simulink model "discrete_model"  (R2018a)
settings: Solver=VariableStepAuto  StartTime=0.0  StopTime=24*60*60  RelTol=1e-3
values from neighbouring files (symbols this model uses):
  alpha = 0.05    [init.m]
  C_T = 12000    [init.m]
  epsilon = 5e-5    (= 5e-05)    [init.m]
  k_N = 2e-4    (= 0.0002)    [init.m]
  k_T = 20    [init.m]
  L0 = 1    [init.m]
  L_opt = 10    [init.m]
  N0 = 1    [init.m]
  N_opt = 150    [init.m]
  q_p = 0.002    [init.m]
  T0 = 20    [init.m]
  T_opt = 22    [init.m]
  T_sample = 1    [init.m]
libraries: simulink x2
settings Model: Creator=Mahsa  LastModifiedBy=Mahsa

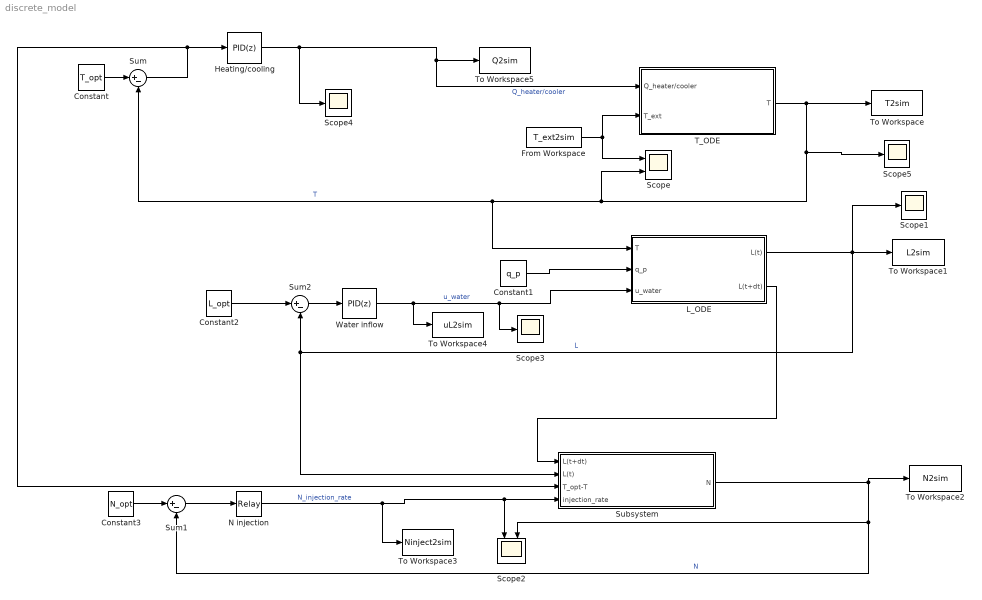
== system discrete_model ==
  Constant : Constant  Value=T_opt
  Constant1 : Constant  Value=q_p
  Constant2 : Constant  Value=L_opt
  Constant3 : Constant  Value=N_opt
  From Workspace : FromWorkspace  VariableName=T_ext2sim  SampleTime=0
  "Heating/cooling " : simulink/Continuous/PID Controller  Controller=PID  TimeDomain=Discrete-time  SampleTime=T_sample  IntegratorMethod=Forward Euler  FilterMethod=Forward Euler  Form=Parallel  UseFilter=on  ControllerParametersSource=internal  P=26.6328130643636  I=0.0891686910196959  D=-511.482477785438  N=0.00506771888250834  InitialConditionSource=internal  InitialConditionForIntegrator=0  InitialConditionForFilter=0  ExternalReset=none  LimitOutput=off  UpperSaturationLimit=inf  LowerSaturationLimit=-inf  LinearizeAsGain=on  AntiWindupMode=none  Kb=1  TrackingMode=off  Kt=1  PParamMin=[]  PParamMax=[]  IParamMin=[]  IParamMax=[]  DParamMin=[]  DParamMax=[]  NParamMin=[]  NParamMax=[]  KbParamMin=[]  KbParamMax=[]  KtParamMin=[]  KtParamMax=[]  POutMin=[]  POutMax=[]  IOutMin=[]  IOutMax=[]  DOutMin=[]  DOutMax=[]  NOutMin=[]  NOutMax=[]  KbOutMin=[]  KbOutMax=[]  KtOutMin=[]  KtOutMax=[]  IntegratorOutMin=[]  IntegratorOutMax=[]  FilterOutMin=[]  FilterOutMax=[]  SumOutMin=[]  SumOutMax=[]  SumI1OutMin=[]  SumI1OutMax=[]  SumI2OutMin=[]  SumI2OutMax=[]  SumI3OutMin=[]  SumI3OutMax=[]  SumDOutMin=[]  SumDOutMax=[]  SaturationOutMin=[]  SaturationOutMax=[]  IntegratorContinuousStateAttributes=''  IntegratorStateMustResolveToSignalObject=off  IntegratorRTWStateStorageClass=Auto  FilterContinuousStateAttributes=''  FilterStateMustResolveToSignalObject=off  FilterRTWStateStorageClass=Auto  DifferentiatorICPrevScaledInput=0  DifferentiatorOutMin=[]  DifferentiatorOutMax=[]  FilterDiffOutCoefMin=[]  FilterDiffOutCoefMax=[]  SumDenOutMin=[]  SumDenOutMax=[]  SumNumOutMin=[]  SumNumOutMax=[]  ReciprocalOutMin=[]  ReciprocalOutMax=[]  DivideOutMin=[]  DivideOutMax=[]  TunerSelectOption=Transfer Function Based (PID Tuner App)
  L_ODE : Subsystem
  N injection : Relay  OnSwitchValue=50  OffSwitchValue=-50  OnOutputValue=R
  Scope : Scope  NumInputPorts=2
  Scope{1,3..5} (4 alike) : Scope
  Scope2 : Scope  NumInputPorts=2
  Subsystem : Subsystem
  Sum : Sum  Inputs=|+-
  Sum1 : Sum  Inputs=|+-
  Sum2 : Sum  Inputs=|+-
  T_ODE : Subsystem
  To Workspace : ToWorkspace  VariableName=T2sim  SaveFormat=Timeseries  SampleTime=T_sample
  To Workspace1 : ToWorkspace  VariableName=L2sim  SaveFormat=Timeseries  SampleTime=T_sample
  To Workspace2 : ToWorkspace  VariableName=N2sim  SaveFormat=Timeseries  SampleTime=T_sample
  To Workspace3 : ToWorkspace  VariableName=Ninject2sim  SaveFormat=Timeseries  SampleTime=T_sample
  To Workspace4 : ToWorkspace  VariableName=uL2sim  SaveFormat=Timeseries  SampleTime=T_sample
  To Workspace5 : ToWorkspace  VariableName=Q2sim  SaveFormat=Timeseries  SampleTime=T_sample
  Water inflow : simulink/Continuous/PID Controller  Controller=PID  TimeDomain=Discrete-time  SampleTime=T_sample  IntegratorMethod=Forward Euler  FilterMethod=Forward Euler  Form=Parallel  UseFilter=on  ControllerParametersSource=internal  P=0.028808901415482  I=0.000153529168152366  D=-0.200332739399639  N=0.0470716938872077  InitialConditionSource=internal  InitialConditionForIntegrator=0  InitialConditionForFilter=0  ExternalReset=none  LimitOutput=on  UpperSaturationLimit=inf  LowerSaturationLimit=0  LinearizeAsGain=on  AntiWindupMode=none  Kb=1  TrackingMode=off  Kt=1  PParamMin=[]  PParamMax=[]  IParamMin=[]  IParamMax=[]  DParamMin=[]  DParamMax=[]  NParamMin=[]  NParamMax=[]  KbParamMin=[]  KbParamMax=[]  KtParamMin=[]  KtParamMax=[]  POutMin=[]  POutMax=[]  IOutMin=[]  IOutMax=[]  DOutMin=[]  DOutMax=[]  NOutMin=[]  NOutMax=[]  KbOutMin=[]  KbOutMax=[]  KtOutMin=[]  KtOutMax=[]  IntegratorOutMin=[]  IntegratorOutMax=[]  FilterOutMin=[]  FilterOutMax=[]  SumOutMin=[]  SumOutMax=[]  SumI1OutMin=[]  SumI1OutMax=[]  SumI2OutMin=[]  SumI2OutMax=[]  SumI3OutMin=[]  SumI3OutMax=[]  SumDOutMin=[]  SumDOutMax=[]  SaturationOutMin=[]  SaturationOutMax=[]  IntegratorContinuousStateAttributes=''  IntegratorStateMustResolveToSignalObject=off  IntegratorRTWStateStorageClass=Auto  FilterContinuousStateAttributes=''  FilterStateMustResolveToSignalObject=off  FilterRTWStateStorageClass=Auto  DifferentiatorICPrevScaledInput=0  DifferentiatorOutMin=[]  DifferentiatorOutMax=[]  FilterDiffOutCoefMin=[]  FilterDiffOutCoefMax=[]  SumDenOutMin=[]  SumDenOutMax=[]  SumNumOutMin=[]  SumNumOutMax=[]  ReciprocalOutMin=[]  ReciprocalOutMax=[]  DivideOutMin=[]  DivideOutMax=[]  TunerSelectOption=Transfer Function Based (PID Tuner App)
  wires:
  Sum1/1 -> N injection/1
  Sum2/1 -> Water inflow/1
  T_ODE/1(T) -> Scope5/1, Scope/2, L_ODE/1(T), Sum/2, To Workspace/1  "T"
  "Heating/cooling "/1 -> Scope4/1, To Workspace5/1, T_ODE/1(Q_heater/cooler)  "Q_heater/cooler"
  Constant/1 -> Sum/1
  From Workspace/1 -> Scope/1, T_ODE/2(T_ext)
  Constant2/1 -> Sum2/1
  Water inflow/1 -> To Workspace4/1, Scope3/1, L_ODE/3(u_water)  "u_water"
  Constant1/1 -> L_ODE/2(q_p)
  L_ODE/1(L(t)) -> Subsystem/2(L(t)), Sum2/2, Scope1/1, To Workspace1/1  "L"
  Constant3/1 -> Sum1/1
  Subsystem/1("N ") -> To Workspace2/1, Sum1/2, Scope2/2  "N"
  L_ODE/2(L(t+dt)) -> Subsystem/1(L(t+dt))
  N injection/1 -> To Workspace3/1, Scope2/1, Subsystem/4(injection_rate)  "N_injection_rate"
  Sum/1 -> Subsystem/3(T_opt-T), "Heating/cooling "/1

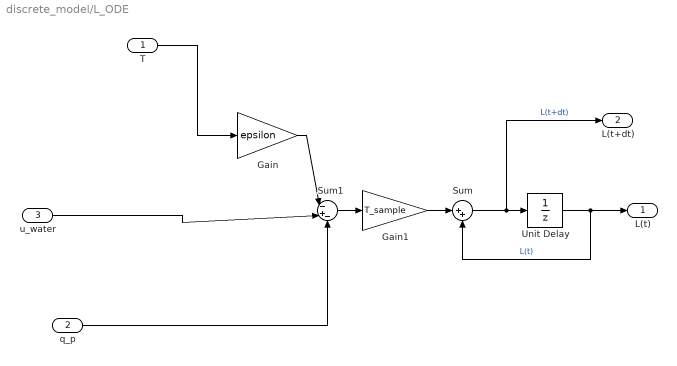
== system discrete_model/L_ODE ==
  T : Inport
  q_p : Inport  Port=2
  u_water : Inport  Port=3
  Gain : Gain  Gain=epsilon
  Gain1 : Gain  Gain=T_sample
  Sum : Sum  Inputs=|++
  Sum1 : Sum  Inputs=|-+-
  Unit Delay : UnitDelay  InitialCondition=L0  SampleTime=T_sample
  L(t) : Outport
  L(t+dt) : Outport  Port=2
  wires:
  Sum1/1 -> Gain1/1
  T/1 -> Gain/1
  Gain/1 -> Sum1/1
  u_water/1 -> Sum1/2
  q_p/1 -> Sum1/3
  Unit Delay/1 -> Sum/2, L(t)/1  "L(t)"
  Gain1/1 -> Sum/1
  Sum/1 -> L(t+dt)/1, Unit Delay/1  "L(t+dt)"

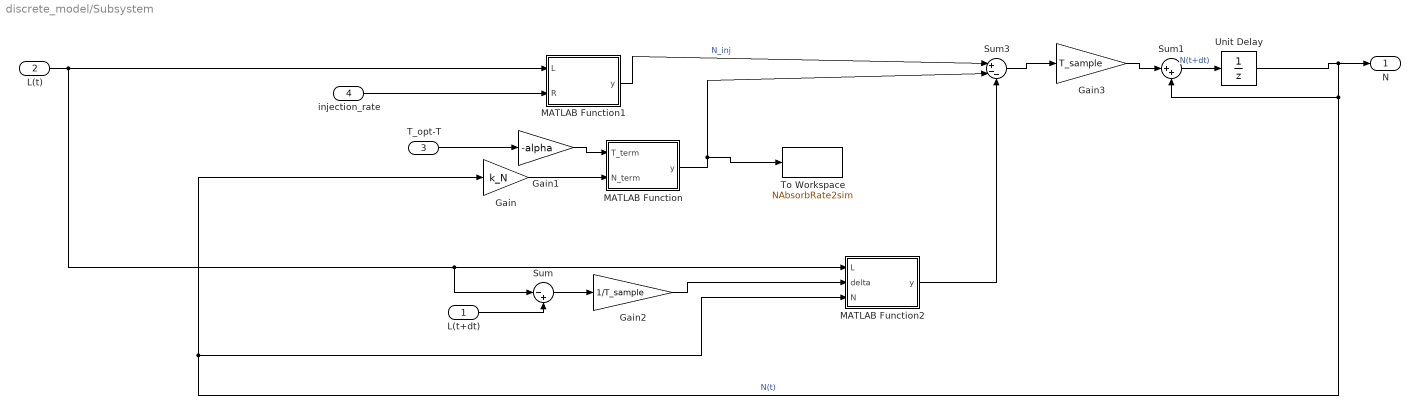
== system discrete_model/Subsystem ==
  L(t+dt) : Inport
  L(t) : Inport  Port=2
  T_opt-T : Inport  Port=3
  injection_rate : Inport  Port=4
  Gain : Gain  Gain=k_N
  Gain1 : Gain  Gain=-alpha
  Gain2 : Gain  Gain=1/T_sample
  Gain3 : Gain  Gain=T_sample
  MATLAB Function : MATLAB Function  TreatAsAtomicUnit=on
  MATLAB Function1 : MATLAB Function  TreatAsAtomicUnit=on
  MATLAB Function2 : MATLAB Function  TreatAsAtomicUnit=on
  Sum : Sum  Inputs=|-+
  Sum1 : Sum  Inputs=|++
  Sum3 : Sum  Inputs=|+--
  To Workspace : ToWorkspace  VariableName=NAbsorbRate2sim  SaveFormat=Timeseries  SampleTime=T_sample
  Unit Delay : UnitDelay  InitialCondition=N0  SampleTime=T_sample
  "N " : Outport
  wires:
  MATLAB Function2/1(y) -> Sum3/3
  MATLAB Function1/1(y) -> Sum3/1  "N_inj"
  MATLAB Function/1(y) -> To Workspace/1, Sum3/2
  injection_rate/1 -> MATLAB Function1/2(R)
  Gain/1 -> MATLAB Function/2(N_term)
  Gain1/1 -> MATLAB Function/1(T_term)
  L(t)/1 -> Sum/1, MATLAB Function2/1(L), MATLAB Function1/1(L)
  T_opt-T/1 -> Gain1/1
  Unit Delay/1 -> Gain/1, MATLAB Function2/3(N), Sum1/2, "N "/1  "N(t)"
  L(t+dt)/1 -> Sum/2
  Sum/1 -> Gain2/1
  Gain2/1 -> MATLAB Function2/2(delta)
  Sum3/1 -> Gain3/1
  Gain3/1 -> Sum1/1
  Sum1/1 -> Unit Delay/1  "N(t+dt)"

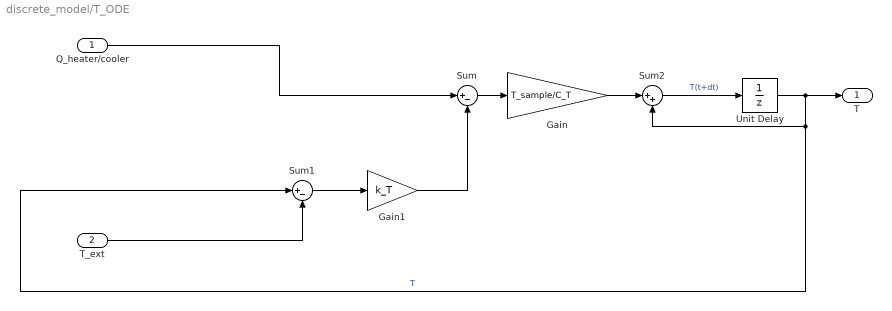
== system discrete_model/T_ODE ==
  Q_heater/cooler : Inport
  T_ext : Inport  Port=2
  Gain : Gain  Gain=T_sample/C_T
  Gain1 : Gain  Gain=k_T
  Sum : Sum  Inputs=|+-
  Sum1 : Sum  Inputs=|+-
  Sum2 : Sum  Inputs=|++
  Unit Delay : UnitDelay  InitialCondition=T0  SampleTime=T_sample
  T : Outport
  wires:
  Gain/1 -> Sum2/1
  T_ext/1 -> Sum1/2
  Sum1/1 -> Gain1/1
  Gain1/1 -> Sum/2
  Unit Delay/1 -> Sum1/1, Sum2/2, T/1  "T"
  Q_heater/cooler/1 -> Sum/1
  Sum/1 -> Gain/1
  Sum2/1 -> Unit Delay/1  "T(t+dt)"

== matlab function discrete_model/Subsystem/MATLAB Function1 ==
  data: L input; y output; R input
function y = fcn(L,R)

y = R./L;

== matlab function discrete_model/Subsystem/MATLAB Function ==
  data: T_term input; y output; N_term input
function y = fcn(T_term,N_term)

y = N_term.*(1+T_term);

== matlab function discrete_model/Subsystem/MATLAB Function2 ==
  data: L input; y output; delta input; N input
function y = fcn(L,delta,N)

y = delta.*N./L;
